simulink model "hyperjack"  (R2021a)
settings: Solver=ode1  StartTime=0.0  StopTime=10.0  FixedStep=0.01  RelTol=1e-3
settings Model: Creator=lilic  LastModifiedBy=Jieming

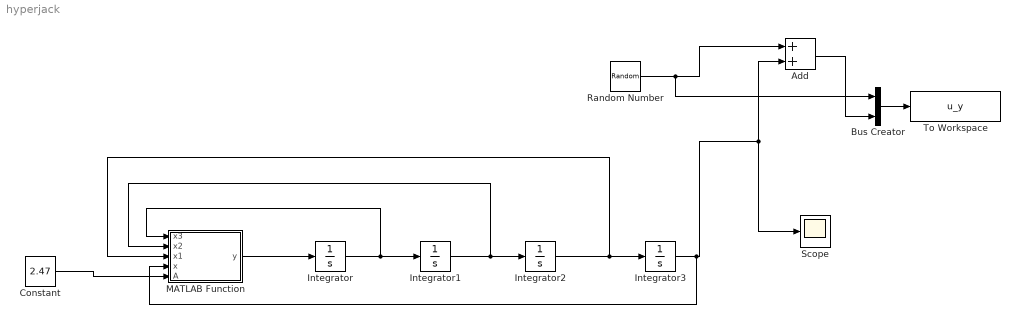
== system hyperjack ==
  Add : Sum
  Bus Creator : BusCreator  Inputs=2
  Constant : Constant  Value=2.47
  Integrator : Integrator  InitialCondition=-0.11
  Integrator1 : Integrator  InitialCondition=-0.55
  Integrator2 : Integrator  InitialCondition=0.5
  Integrator3 : Integrator  InitialCondition=0.01
  MATLAB Function : MATLAB Function  TreatAsAtomicUnit=on
  Random Number : RandomNumber  Variance=0
  Scope : Scope
  To Workspace : ToWorkspace  VariableName=u_y  SaveFormat=Timeseries  SampleTime=-1
  wires:
  Integrator/1 -> MATLAB Function/1(x3), Integrator1/1
  MATLAB Function/1(y) -> Integrator/1
  Bus Creator/1 -> To Workspace/1
  Integrator3/1 -> MATLAB Function/4(x), Add/2, Scope/1
  Integrator2/1 -> MATLAB Function/3(x1), Integrator3/1
  Constant/1 -> MATLAB Function/5(A)
  Integrator1/1 -> MATLAB Function/2(x2), Integrator2/1
  Random Number/1 -> Bus Creator/1, Add/1
  Add/1 -> Bus Creator/2

== matlab function hyperjack/MATLAB Function ==
  data: x3 input; x2 input; x1 input; y output; x input; A input
function y = fcn(x3,x2,x1,x,A)
y = -(x3+A*x2+x1-(x^2-1));
